simulink library "INT_MRly_ShOff"  (R2016b)
settings: Solver=VariableStepAuto  StartTime=0.0  StopTime=10.0  RelTol=1e-3
settings Model: Creator=Administrator  LastModifiedBy=Administrator

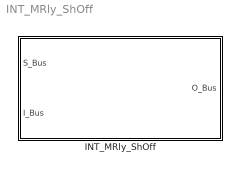
== system INT_MRly_ShOff ==
  INT_MRly_ShOff : Subsystem

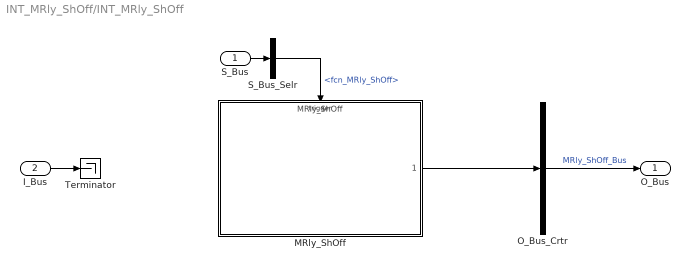
== system INT_MRly_ShOff/INT_MRly_ShOff ==
  S_Bus : Inport
  I_Bus : Inport  Port=2
  MRly_ShOff : ModelReference  ModelNameDialog=MRly_ShOff  SimulationMode=Normal  ModelReferenceVersion=1.2  TriggerPortName=function  TriggerPortTriggerType=function-call  TriggerPortStatesWhenEnabling=held
  O_Bus_Crtr : BusCreator  Inputs=1
  S_Bus_Selr : BusSelector  OutputSignals=fcn_MRly_ShOff
  Terminator : Terminator
  O_Bus : Outport
  wires:
  S_Bus_Selr/1 -> MRly_ShOff/Trigger  "<fcn_MRly_ShOff>"
  S_Bus/1 -> S_Bus_Selr/1
  I_Bus/1 -> Terminator/1
  O_Bus_Crtr/1 -> O_Bus/1  "MRly_ShOff_Bus"
  MRly_ShOff/1 -> O_Bus_Crtr/1
